simulink model "a_T_vector_tgo_iterator_v1"  (R2016b)
settings: Solver=VariableStepAuto  StartTime=0.0  StopTime=70  RelTol=1e-3
values from neighbouring files (symbols this model uses):
  m0 = 58000    [E_Guidance_Modular.m]    (also in E_Guidance_Wong.m; E_Guidance_advanced.m; E_Guidance_advanced_hybrid.m; E_Guidance_advanced_thrust_optimization.m)
  mu = 4.282828185603917*10^13    (= 4.2828281856e+13)    [E_Guidance_Modular.m]    (also in E_Guidance_Wong.m; E_Guidance_advanced.m; E_Guidance_advanced_hybrid.m; E_Guidance_advanced_thrust_optimization.m)
  r0 = A*r0    [E_Guidance_Modular.m]    (also in E_Guidance_Wong.m; E_Guidance_advanced.m; E_Guidance_advanced_hybrid.m; E_Guidance_advanced_thrust_optimization.m)
  rf = A*rf    [E_Guidance_Modular.m]    (also in E_Guidance_Wong.m; E_Guidance_advanced.m; E_Guidance_advanced_hybrid.m; E_Guidance_advanced_thrust_optimization.m)
  rtol = 10    [E_Guidance_sim.m]
  T_max = 800000    [E_Guidance_Modular.m]    (also in E_Guidance_Wong.m; E_Guidance_advanced.m; E_Guidance_advanced_hybrid.m; E_Guidance_advanced_thrust_optimization.m)
  T_min = 200000    [E_Guidance_Modular.m]    (also in E_Guidance_Wong.m; E_Guidance_advanced.m; E_Guidance_advanced_hybrid.m; E_Guidance_advanced_thrust_optimization.m)
  tol_tgo = 0.01    [E_Guidance_sim.m]
  V0 = A*V0    [E_Guidance_Modular.m]    (also in E_Guidance_Wong.m; E_Guidance_advanced.m; E_Guidance_advanced_hybrid.m; E_Guidance_advanced_thrust_optimization.m)
  v_ex = 3531.7    [E_Guidance_Modular.m]    (also in E_Guidance_Wong.m; E_Guidance_advanced.m; E_Guidance_advanced_hybrid.m; E_Guidance_advanced_thrust_optimization.m)
  Vf = A*Vf    [E_Guidance_Modular.m]    (also in E_Guidance_Wong.m; E_Guidance_advanced.m; E_Guidance_advanced_hybrid.m; E_Guidance_advanced_thrust_optimization.m)
libraries: simulink x1
settings Model: Creator=lloyd.strohl  LastModifiedBy=lloyd.strohl

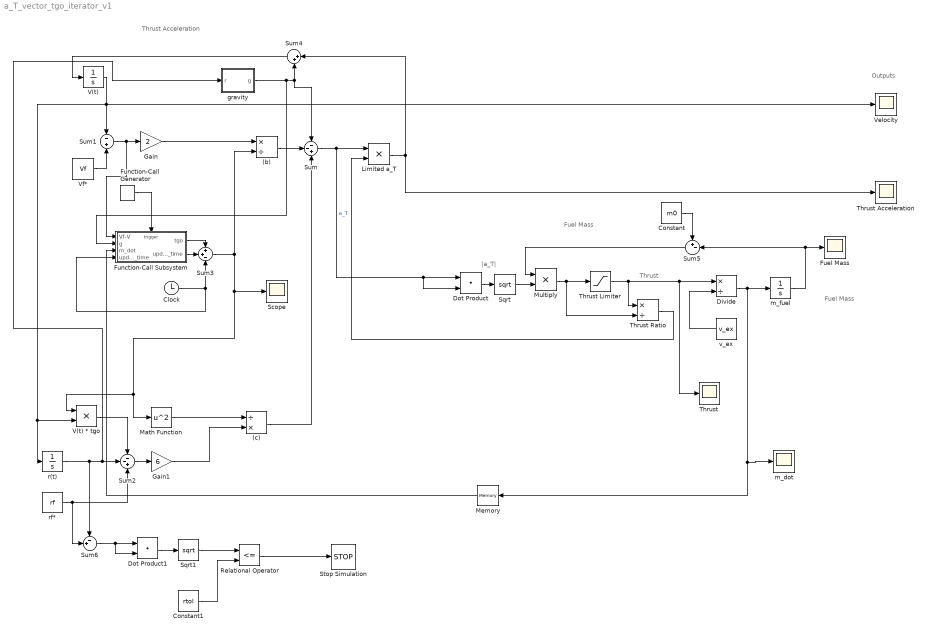
== system a_T_vector_tgo_iterator_v1 ==
  note: Fuel Mass
  note: Thrust
  note: Fuel Mass
  note: Outputs
  note: Thrust Acceleration
  note: |a_T|
  (b) : Product  Inputs=*/
  (c) : Product  Inputs=/*
  Clock : Clock
  Constant : Constant  Value=m0
  Constant1 : Constant  Value=rtol
  Divide : Product  Inputs=*/
  Dot Product : DotProduct  InputSameDT=on  OutDataTypeStr=Inherit: Inherit via internal rule
  Dot Product1 : DotProduct  InputSameDT=on  OutDataTypeStr=Inherit: Inherit via internal rule
  Fuel Mass : Scope
  Function-Call Generator : simulink/Ports & Subsystems/Function-Call Generator  sample_time=1  numberOfIterations=1
  Function-Call Subsystem : Subsystem  TreatAsAtomicUnit=on
  Gain : Gain  Gain=2
  Gain1 : Gain  Gain=6
  Limited a_T : Product  Inputs=**
  Math Function : Math  Operator=square  SaturateOnIntegerOverflow=on
  Memory : Memory  X0=T_max / v_ex
  Multiply : Product
  Relational Operator : RelationalOperator  Operator=<=  OutDataTypeStr=boolean  RndMeth=Simplest
  Scope : Scope
  Sqrt : Sqrt  SaturateOnIntegerOverflow=on
  Sqrt1 : Sqrt  SaturateOnIntegerOverflow=on
  Stop Simulation : Stop
  Sum : Sum  Inputs=--+
  Sum1 : Sum  Inputs=-+
  Sum2 : Sum  Inputs=--+
  Sum3 : Sum  Inputs=++-
  Sum4 : Sum  Inputs=|++
  Sum5 : Sum  Inputs=+-|
  Sum6 : Sum  Inputs=-+|
  Thrust : Scope
  Thrust Acceleration : Scope
  Thrust Limiter : Saturate  UpperLimit=T_max  LowerLimit=T_min
  Thrust Ratio : Product  Inputs=*/
  V(t) : Integrator  InitialCondition=V0  ContinuousStateAttributes='Velocity'
  V(t) * tgo : Product
  Velocity : Scope
  Vf* : Constant  Value=Vf
  gravity : Subsystem
  m_dot : Scope
  m_fuel : Integrator  ContinuousStateAttributes='Fuel_Mass'
  r(t) : Integrator  InitialCondition=r0  ContinuousStateAttributes='Position'
  rf* : Constant  Value=rf
  v_ex : Constant  Value=v_ex
  wires:
  gravity/1(g) -> Function-Call Subsystem/2("g "), Sum4/2, Sum/1
  r(t)/1 -> Sum2/2, gravity/1(r), Sum6/1
  V(t)/1 -> Velocity/1, Sum1/1, V(t) * tgo/2, r(t)/1
  (b)/1 -> Sum/2
  Sum1/1 -> Function-Call Subsystem/1(" Vf-V "), Gain/1
  Gain/1 -> (b)/1
  Sum2/1 -> Gain1/1
  Gain1/1 -> (c)/2
  Math Function/1 -> (c)/1
  (c)/1 -> Sum/3
  rf*/1 -> Sum2/3, Sum6/2
  V(t) * tgo/1 -> Sum2/1
  Vf*/1 -> Sum1/2
  Sqrt/1 -> Multiply/2
  v_ex/1 -> Divide/2
  Divide/1 -> m_dot/1, Memory/1, m_fuel/1
  m_fuel/1 -> Fuel Mass/1, Sum5/2
  Sum4/1 -> V(t)/1
  Sum5/1 -> Multiply/1
  Constant/1 -> Sum5/1
  Dot Product/1 -> Sqrt/1
  Multiply/1 -> Thrust Ratio/2, Thrust Limiter/1
  Thrust Limiter/1 -> Thrust Ratio/1, Divide/1, Thrust/1
  Sum/1 -> Limited a_T/1, Dot Product/2, Dot Product/1  "a_T"
  Thrust Ratio/1 -> Limited a_T/2
  Limited a_T/1 -> Sum4/1, Thrust Acceleration/1
  Function-Call Generator/1 -> Function-Call Subsystem/Trigger
  Clock/1 -> Sum3/3, Function-Call Subsystem/4(update_time)
  Function-Call Subsystem/2("update_time ") -> Sum3/2
  Function-Call Subsystem/1(tgo) -> Sum3/1
  Sum3/1 -> Math Function/1, V(t) * tgo/1, Scope/1, (b)/2
  Memory/1 -> Function-Call Subsystem/3("m_dot ")
  Sum6/1 -> Dot Product1/1, Dot Product1/2
  Dot Product1/1 -> Sqrt1/1
  Constant1/1 -> Relational Operator/2
  Sqrt1/1 -> Relational Operator/1
  Relational Operator/1 -> Stop Simulation/1

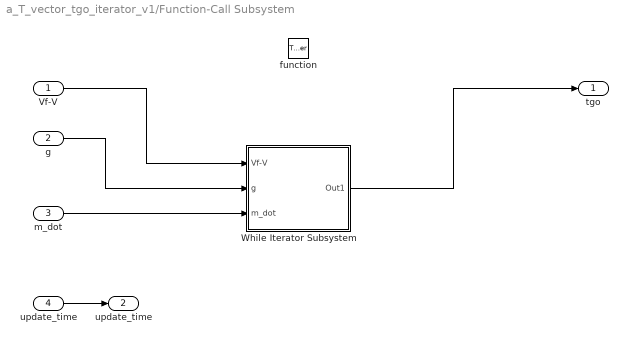
== system a_T_vector_tgo_iterator_v1/Function-Call Subsystem ==
  " Vf-V " : Inport
  "g " : Inport  Port=2
  "m_dot " : Inport  Port=3
  update_time : Inport  Port=4
  function : TriggerPort  TriggerType=function-call  VariantControl=Variant
  While Iterator Subsystem : Subsystem  TreatAsAtomicUnit=on
  tgo : Outport  SourceOfInitialOutputValue=Input signal  OutputWhenDisabled=reset  InitialOutput=0
  "update_time " : Outport  Port=2  SourceOfInitialOutputValue=Input signal  OutputWhenDisabled=reset  InitialOutput=0
  wires:
  " Vf-V "/1 -> While Iterator Subsystem/1(Vf-V)
  "g "/1 -> While Iterator Subsystem/2(g)
  While Iterator Subsystem/1(Out1) -> tgo/1
  update_time/1 -> "update_time "/1
  "m_dot "/1 -> While Iterator Subsystem/3(m_dot)

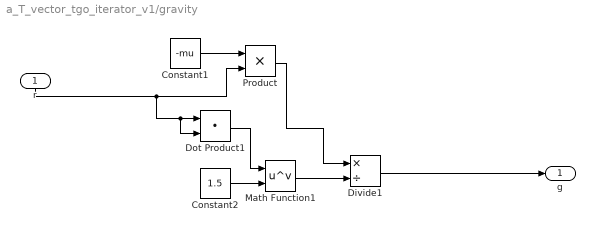
== system a_T_vector_tgo_iterator_v1/gravity ==
  r : Inport
  Constant1 : Constant  Value=-mu
  Constant2 : Constant  Value=1.5
  Divide1 : Product  Inputs=*/
  Dot Product1 : DotProduct  InputSameDT=on  OutDataTypeStr=Inherit: Inherit via internal rule
  Math Function1 : Math  Operator=pow  SaturateOnIntegerOverflow=on
  Product : Product
  g : Outport
  wires:
  r/1 -> Product/2, Dot Product1/2, Dot Product1/1
  Math Function1/1 -> Divide1/2
  Product/1 -> Divide1/1
  Constant2/1 -> Math Function1/2
  Constant1/1 -> Product/1
  Dot Product1/1 -> Math Function1/1
  Divide1/1 -> g/1

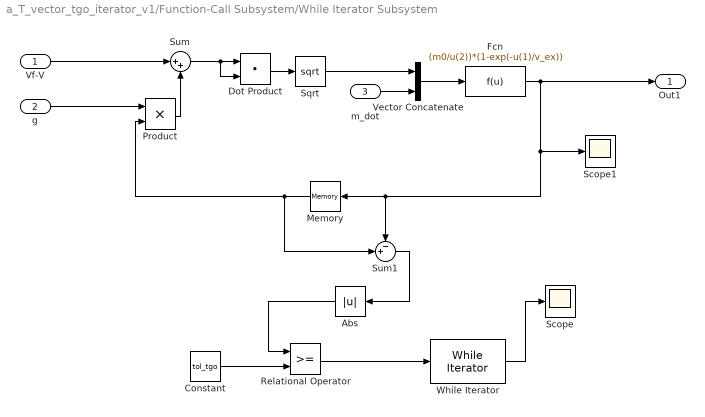
== system a_T_vector_tgo_iterator_v1/Function-Call Subsystem/While Iterator Subsystem ==
  Vf-V : Inport
  g : Inport  Port=2
  m_dot : Inport  Port=3
  Abs : Abs
  Constant : Constant  Value=tol_tgo
  Dot Product : DotProduct  InputSameDT=on  OutDataTypeStr=Inherit: Inherit via internal rule
  Fcn : Fcn  Expr=(m0/u(2))*(1-exp(-u(1)/v_ex))
  Memory : Memory  X0=60  InheritSampleTime=on
  Product : Product
  Relational Operator : RelationalOperator  OutDataTypeStr=boolean  RndMeth=Simplest
  Scope : Scope
  Scope1 : Scope
  Sqrt : Sqrt  SaturateOnIntegerOverflow=on
  Sum : Sum  Inputs=|++
  Sum1 : Sum  Inputs=-+|
  Vector Concatenate : Concatenate
  While Iterator : WhileIterator  MaxIters=20  WhileBlockType=do-while  ShowIterationPort=on
  Out1 : Outport
  wires:
  g/1 -> Product/1
  Vf-V/1 -> Sum/1
  Product/1 -> Sum/2
  Sum/1 -> Dot Product/2, Dot Product/1
  Dot Product/1 -> Sqrt/1
  m_dot/1 -> Vector Concatenate/2
  Sqrt/1 -> Vector Concatenate/1
  Vector Concatenate/1 -> Fcn/1
  Memory/1 -> Sum1/2, Product/2
  Fcn/1 -> Scope1/1, Sum1/1, Memory/1, Out1/1
  Constant/1 -> Relational Operator/2
  Abs/1 -> Relational Operator/1
  Relational Operator/1 -> While Iterator/1
  Sum1/1 -> Abs/1
  While Iterator/1 -> Scope/1
